simulink model "Controle_MPC_AviaoITAE"  (R2025b)
settings: Solver=VariableStepAuto  StartTime=0.0  StopTime=10.0  RelTol=1e-3
libraries: cstblocks x1, mpclib x1
settings Model: Creator=felip

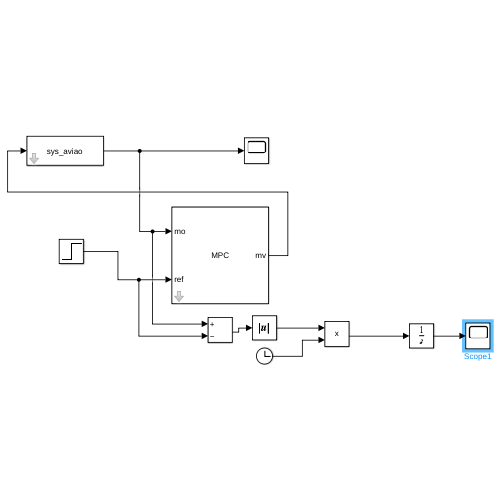
[thumbnail: Simulink's stored preview of the top-level diagram]
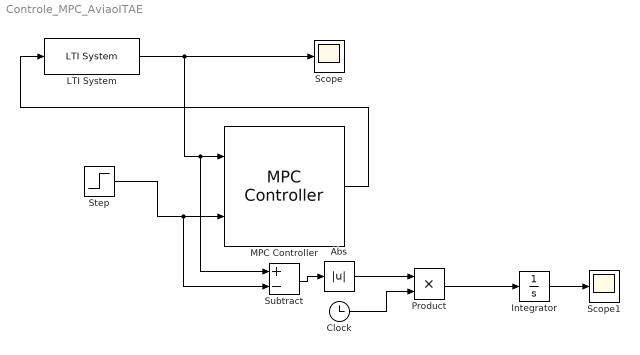
== system Controle_MPC_AviaoITAE ==
  Abs : Abs  SaturateOnIntegerOverflow=off
  Clock : Clock
  Integrator : Integrator
  LTI System : cstblocks/LTI System  sys=sys_aviao  IC=[]  PadeOrder=0
  MPC Controller : mpclib/MPC Controller  SCDEnableBlockLinearizationSpecification=on  mpcobj=mpc1  is_multiple=0  enable_value=0  return_u0=off  updateMPCinCallerWorkspace=on  md_inport=off  mv_inport=off  uref_inport=off  return_cost=off  return_mvseq=off  return_qpstatus=off  return_xseq=off  return_state=off  return_ovseq=off  state_inport=off  umin_inport=off  umax_inport=off  ymin_inport=off  ymax_inport=off  cc_inport=off  ywt_inport=off  uwt_inport=off  duwt_inport=off  rhoeps_inport=off  pm_inport=off  MaximumP=10  HorizonChoice=FixedHorizon  n_ts=0.1  n_p=10  n_mv=1  n_md=0  n_ud=0  n_mo=1  n_uo=0  BlockDataType=double  SampleTimeInherited=off  switch_inport=off
  Product : Product
  Scope : Scope
      settings: ActiveDisplayYMinimum=-0.11254963995084988  ActiveDisplayYMaximum=0.35155156706727242
  Scope1 : Scope
      settings: ActiveDisplayYMinimum=-0.43789815586241543  ActiveDisplayYMaximum=0.81240805735037436
  Step : Step  After=0.2  SampleTime=0
  Subtract : Sum  Inputs=+-
  wires:
  Product/1 -> Integrator/1
  LTI System/1 -> Subtract/1, MPC Controller/1, Scope/1
  Step/1 -> Subtract/2, MPC Controller/2
  MPC Controller/1 -> LTI System/1
  Subtract/1 -> Abs/1
  Integrator/1 -> Scope1/1
  Abs/1 -> Product/1
  Clock/1 -> Product/2
